simulink library "SafetyCheckerSOMANET"  (R2016b)
settings: Solver=VariableStepAuto  StartTime=0.0  StopTime=10.0  RelTol=1e-3
libraries: I2tChecker x1, PhaseCurrentsChecker x1, TemperatureSomanetChecker x1, TimestampChecker x1, TorqueChecker x1
settings Model: Creator=Nathan  LastModifiedBy=MARCH

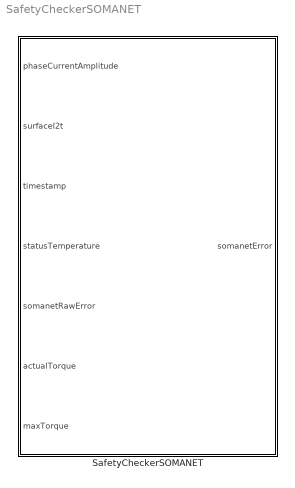
== system SafetyCheckerSOMANET ==
  SafetyCheckerSOMANET : Subsystem

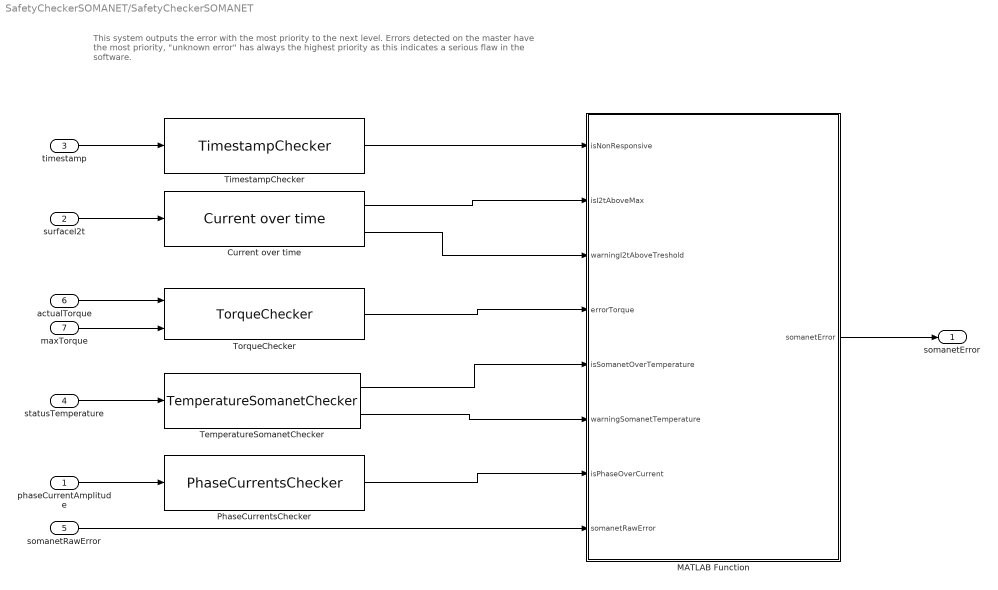
== system SafetyCheckerSOMANET/SafetyCheckerSOMANET ==
  note: This system outputs the error with the most priority to the next level.
      | Errors detected on the master have the most priority, "unknown error" has always the highest priority as this indicates a serious flaw in the software.
  phaseCurrentAmplitude : Inport
  surfaceI2t : Inport  Port=2
  timestamp : Inport  Port=3  BusOutputAsStruct=on
  statusTemperature : Inport  Port=4  BusOutputAsStruct=on
  somanetRawError : Inport  Port=5
  actualTorque : Inport  Port=6
  maxTorque : Inport  Port=7
  Current over time : I2tChecker/Current over time
  MATLAB Function : MATLAB Function  TreatAsAtomicUnit=on
  PhaseCurrentsChecker : PhaseCurrentsChecker/PhaseCurrentsChecker
  TemperatureSomanetChecker : TemperatureSomanetChecker/TemperatureSomanetChecker
  TimestampChecker : TimestampChecker/TimestampChecker
  TorqueChecker : TorqueChecker/TorqueChecker
  somanetError : Outport
  wires:
  maxTorque/1 -> TorqueChecker/2
  somanetRawError/1 -> MATLAB Function/8(somanetRawError)
  TemperatureSomanetChecker/1 -> MATLAB Function/5(isSomanetOverTemperature)
  PhaseCurrentsChecker/1 -> MATLAB Function/7(isPhaseOverCurrent)
  TemperatureSomanetChecker/2 -> MATLAB Function/6(warningSomanetTemperature)
  TorqueChecker/1 -> MATLAB Function/4(errorTorque)
  Current over time/2 -> MATLAB Function/3(warningI2tAboveTreshold)
  Current over time/1 -> MATLAB Function/2(isI2tAboveMax)
  TimestampChecker/1 -> MATLAB Function/1(isNonResponsive)
  actualTorque/1 -> TorqueChecker/1
  statusTemperature/1 -> TemperatureSomanetChecker/1
  phaseCurrentAmplitude/1 -> PhaseCurrentsChecker/1
  timestamp/1 -> TimestampChecker/1
  MATLAB Function/1(somanetError) -> somanetError/1
  surfaceI2t/1 -> Current over time/1

== matlab function SafetyCheckerSOMANET/MATLAB Function ==
  data: isNonResponsive input; somanetError output; isI2tAboveMax input; warningI2tAboveTreshold input; errorTorque input; isSomanetOverTemperature input; warningSomanetTemperature input; isPhaseOverCurrent input; somanetRawError input
function somanetError = fcn(isNonResponsive,isI2tAboveMax,warningI2tAboveTreshold,errorTorque,isSomanetOverTemperature,warningSomanetTemperature,isPhaseOverCurrent,somanetRawError)

% Errors are in priority
if (somanetRawError == SomanetError.SOMANET_UNKNOWN_ERROR)
    somanetError = SomanetError.SOMANET_UNKNOWN_ERROR;
   
elseif (isNonResponsive ~= 0)
    somanetError = SomanetError.SOMANET_DISCONNECTED;
    
elseif (isI2tAboveMax ~=0)
    somanetError = SomanetError.PHASE_I2T_ERROR;
    
elseif (errorTorque ~=0)
    somanetError = SomanetError.MAX_TORQUE_REACHED;
    
elseif (isSomanetOverTemperature ~= 0)
    somanetError = SomanetError.SOMANET_OVERHEAT;
    
elseif (isPhaseOverCurrent ~= 0)
    somanetError = SomanetError.NOERROR_SOMANET;%SomanetError.PHASE_OVERCURRENT_MASTER_DETECT;
    %this was commented out because it is not necessary. Phase over current
    %is also detected on SOMANET

elseif (somanetRawError ~= SomanetError.NOERROR_SOMANET)
    somanetError = somanetRawError;
    
elseif (warningI2tAboveTreshold ~= 0)
    somanetError = SomanetError.SOMANET_NEAR_I2T_ERROR;
    
elseif (warningSomanetTemperature ~= 0)
    somanetError = SomanetError.SOMANET_NEAR_OVERHEAT;
    
else
    somanetError = SomanetError.NOERROR_SOMANET;
    
end

end
